simulink model "test_freq_fcn"  (R2017b)
settings: Solver=FixedStepDiscrete  StartTime=0.0  StopTime=10*floor(4e-3/Ts)*Ts  FixedStep=Ts  RelTol=1e-3  EnableMultiTasking=on
InitFcn:
  | Fs = 245.76e6;
  | Ts = 1/Fs;
  | Fif = 50e6;
libraries: Library_SignalGeneration x5
settings Model: Creator=Keith  LastModifiedBy=Keith
settings DataIOCC: SaveOutput=off  SignalLogging=off  DSMLogging=off  SaveTime=off
settings OptimizationCC: LifeSpan=inf
settings DebuggingCC: SFUnexpectedBacktrackingDiag=warning  SFNoUnconditionalDefaultTransitionDiag=warning  SFExecutionAtInitializationDiag=none
settings CodeAppCC: StateflowObjectComments=on
settings GRTTargetCC: TargetLangStandard=C89/C90 (ANSI)  GeneratePreprocessorConditionals=Disable all
settings ConfigComp: CovMetricSettings=dw  CovHtmlReporting=on  CovSaveCumulativeToWorkspaceVar=on  CovSaveSingleToWorkspaceVar=on  CovExternalEMLEnable=off

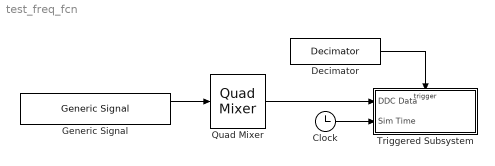
== system test_freq_fcn ==
  Clock : Clock
  Decimator : Library_SignalGeneration/Decimator  parentFs=Fs  decFac=1000
  Generic Signal : Library_SignalGeneration/Generic Signal  fPoints=[20 20]*1e6  dPoints=[20 24]*1e3*0  tPoints=[0 4.0]*1e-3  isPulsed=on  PRF=600e3  PD=.5e-6  FS=245.76e6
  Quad Mixer : Library_SignalGeneration/Quad Mixer  loFrequencyHz=-20e6+40e3
      settings: AttributesFormatString=LO: %<loFrequencyHz>
  Triggered Subsystem : Subsystem  TreatAsAtomicUnit=on
  wires:
  Generic Signal/1 -> Quad Mixer/1
  Quad Mixer/1 -> Triggered Subsystem/1(DDC Data)
  Decimator/1 -> Triggered Subsystem/Trigger
  Clock/1 -> Triggered Subsystem/2(Sim Time)

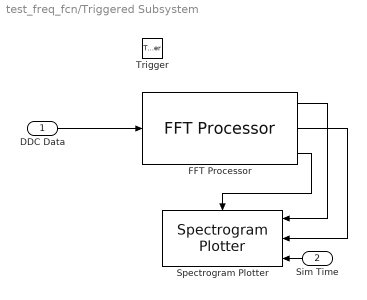
== system test_freq_fcn/Triggered Subsystem ==
  DDC Data : Inport
  Sim Time : Inport  Port=2
  Trigger : TriggerPort  VariantControl=Variant
  FFT Processor : Library_SignalGeneration/FFT Processor  BUFFSIZE=2^8  FFTSIZE=2^8  FOUTRNG=[]  OVLP_PRCNT=0  Fs=Fs/1000  FSCALE=1e-3
  Spectrogram Plotter : Library_SignalGeneration/Spectrogram Plotter  nRows=400  complexFFT=on  Fs=Fs/1000  Zo=50  cMin=-60  cMax=10
      settings: AttributesFormatString=|
      | Fs=%<Fs> | Zo=%<Zo>
      | Displays %<nRows> Rows
  wires:
  FFT Processor/1 -> Spectrogram Plotter/1
  FFT Processor/3 -> Spectrogram Plotter/Trigger
  FFT Processor/2 -> Spectrogram Plotter/2
  Sim Time/1 -> Spectrogram Plotter/3
  DDC Data/1 -> FFT Processor/1
